simulink model "Lab1_parameter_estimation_student"  (R2025b)
settings: Solver=FixedStepAuto  StartTime=0.0  StopTime=inf  FixedStep=0.001  RelTol=1e-3
values from neighbouring files (symbols this model uses):
  motor_B = 0.0001    [Lab1_motor_params_student.m]    (also in R_Squre.m = 0; Validation.m = 2.5762333e-05)
  motor_Eff = 0.5    [Lab1_motor_params_student.m]    (also in R_Squre.m = 0.9668; Validation.m = 0.972957)
  motor_J = 0.001    [Lab1_motor_params_student.m]    (also in R_Squre.m = 1e-05; Validation.m = 1.10153333e-05)
  motor_Ke = 0.05    [Lab1_motor_params_student.m]    (also in R_Squre.m = 0.05161; Validation.m = 0.050013)
  motor_L = 0.01    [Lab1_motor_params_student.m]    (also in R_Squre.m = 0.04016; Validation.m = 0.04016)
  motor_R = 1.00    (= 1)    [Lab1_motor_params_student.m]    (also in R_Squre.m = 3.69; Validation.m = 3.69)
libraries: simulink x1
settings Model: Creator=tanawatp  LastModifiedBy=Akkarasaknarong
settings RTWCC: GPUComputeCapability=3.5

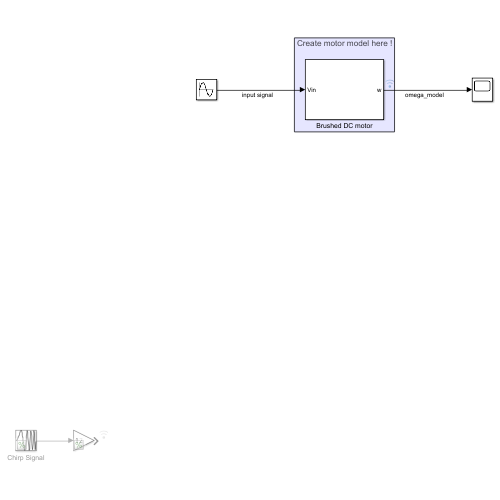
[thumbnail: Simulink's stored preview of the top-level diagram]
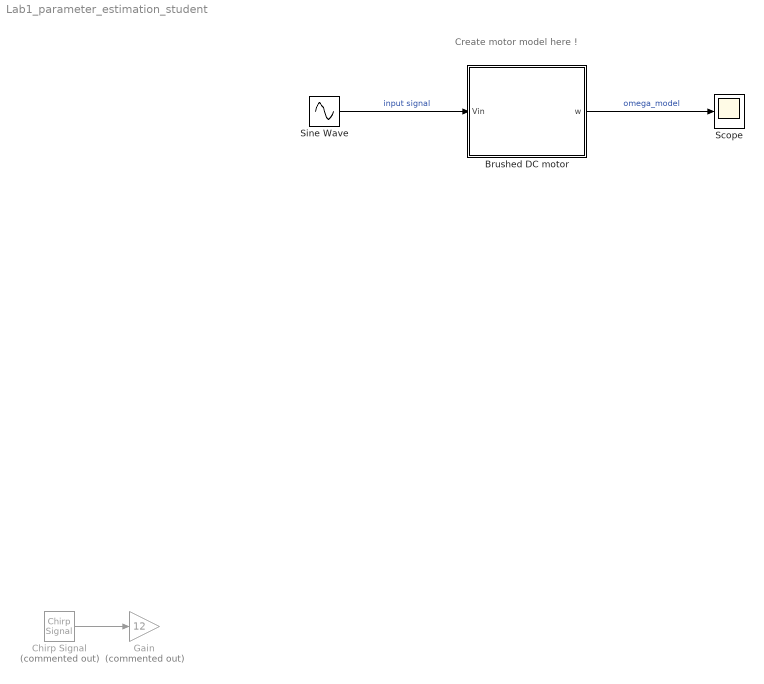
== system Lab1_parameter_estimation_student ==
  note: Create motor model here !
  Brushed DC motor : Subsystem
  Chirp Signal : simulink/Sources/Chirp Signal  Commented=on  f1=0.1  T=40  f2=5
  Gain : Gain  Commented=on  Gain=12
  Scope : Scope
      settings: ActiveDisplayYMinimum=-18.683452593186807  ActiveDisplayYMaximum=18.683452593184636
  Sine Wave : Sin  SampleTime=0
  wires:
  Brushed DC motor/1(w) -> Scope/1  "omega_model"
  Chirp Signal/1 -> Gain/1
  Sine Wave/1 -> Brushed DC motor/1(Vin)  "input signal"

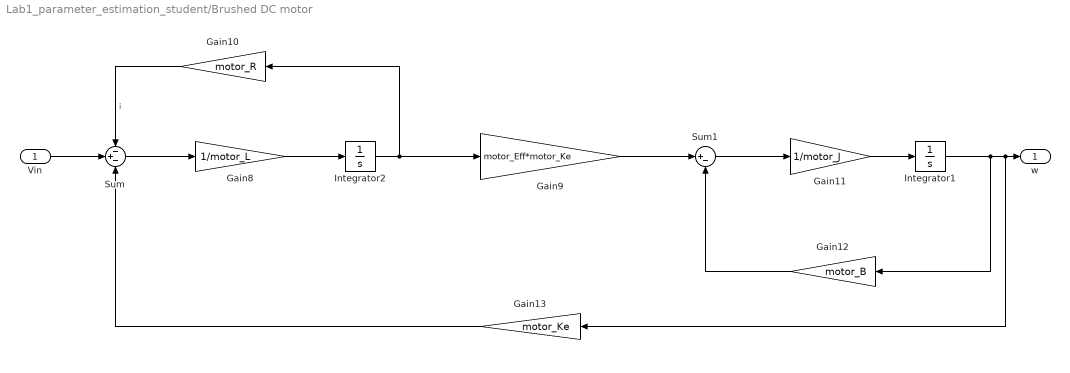
== system Lab1_parameter_estimation_student/Brushed DC motor ==
  Vin : Inport
  Gain10 : Gain  Gain=motor_R
  Gain11 : Gain  Gain=1/motor_J
  Gain12 : Gain  Gain=motor_B
  Gain13 : Gain  Gain=motor_Ke
  Gain8 : Gain  Gain=1/motor_L
  Gain9 : Gain  Gain=motor_Eff*motor_Ke
  Integrator1 : Integrator
  Integrator2 : Integrator
  Sum : Sum  Inputs=-+-
  Sum1 : Sum  Inputs=|+-
  w : Outport
  wires:
  Sum/1 -> Gain8/1
  Gain8/1 -> Integrator2/1
  Integrator2/1 -> Gain9/1, Gain10/1
  Gain10/1 -> Sum/1  "i"
  Vin/1 -> Sum/2
  Gain9/1 -> Sum1/1
  Sum1/1 -> Gain11/1
  Gain11/1 -> Integrator1/1
  Integrator1/1 -> Gain12/1, Gain13/1, w/1
  Gain13/1 -> Sum/3
  Gain12/1 -> Sum1/2
